simulink model "basic_control_structure_kalman"  (Simulink 6.2)
settings: Solver=ode45  StartTime=0.0  StopTime=6174  RelTol=1e-3
libraries: components_lib x12, simulink x5
settings Model: Creator=krage  LastModifiedBy=Martin  ExtModeAutoUpdateStatusClock=off
settings DebuggingCC: CheckSSInitialOutputMsg=off  SolverPrmCheckMsg=warning

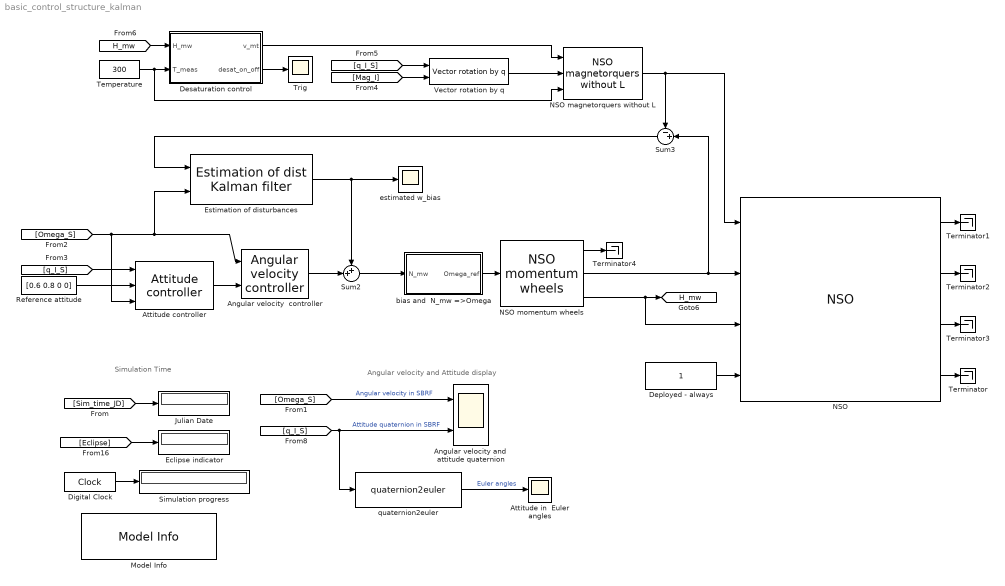
== system basic_control_structure_kalman ==
  note: Simulation Time
  note: Angular velocity and Attitude display
  Angular velocity  controller : components_lib/ACS/Controllers/Angular velocity  controller  ang_file_name='ang_robust_control.m'
  Angular velocity and  attitude quaternion : Scope  NumInputPorts=2
      settings: TimeRange=250  YMin=-0.05~0.1  YMax=0.05~0.9  SaveName=measurement
  Attitude controller : components_lib/ACS/Controllers/Attitude controller  att_file_name='attitude_control_lqr.m'
  Attitude in  Euler angles : Scope
      settings: YMin=-3.5  YMax=3.5
  Deployed - always : Constant
  Desaturation control : Subsystem  mask{h_bias=2.23*1e-3, desat_on=0.7*2.23e-3, desat_off=0.01*2.23e-3}
      mask prompts: h_bias "Angular momentum bias"; desat_on "Threshold desaturation on"; desat_off "Threshold desaturation off"
  Digital Clock : DigitalClock
  Eclipse indicator : Display
  Estimation of disturbances : components_lib/ACS/Controllers/Estimation of dist Kalman filter  ang_file_name='kalman_estimator.m'
  Julian Date : Display
  Model Info : simulink/Model-Wide Utilities/Model Info  InitialBlockCM=None  BlockCM=None  Frame=on  DisplayStringWithTags=|  HorizontalTextAlignment=Left  LeftAlignmentValue=0.02  SourceBlockDiagram=basic_control_structure_kalman  TagMaxNumber=20
      | Usefull Julian dates:
      | sun to eclipse : 2452315.560376
      | 32 sec. before : 2452315.56
      | eclipse to sun : 2452315.513363
  NSO : components_lib/NSO  Tag=AAUSAT-II Model  Description=AAUSAT-II Model  r_com_s=[0.05 0.05 0.15]  sat_temp_start=0  r_com_s_deployed=[0.05 0.05 0.125]  mass_sc=3  Dim=[0.1 0.1 0.3]  inertia_c=[25 25 5]/1e3  inertia_d=[42.3 42.3 28.4]/1e3  init_jd=2452315.56  q_s_c=[0 0 0 1]  q_init_s_i=[0.6 0.8 0 0]  w_init_s=[0.0021 -0.0021 0.0021]*0  Cd=2  rho=9.25e-13  enable_sensor_emulation=off  alb_emu_enabled=off  enable_dist=on
  NSO magnetorquers without L : components_lib/Actuator Emulation/NSO magnetorquers without L
  NSO momentum wheels : components_lib/Actuator Emulation/NSO momentum wheels  w_mw_i=[1078.6 1078.6 1078.6] *0.5
  Reference attitude : Constant  Value=[0.6 0.8 0 0]
  Simulation progress : Display
  Sum2 : Sum  Inputs=++|
  Sum3 : Sum  Orientation=left  Inputs=-+|
  Temperature : Constant  Value=300
  Terminator{,1..4} (5 alike) : Terminator
  Trig : Scope
      settings: YMin=0.95  YMax=1.05  SaveName=ScopeData2
  Vector rotation by q : components_lib/Math utilities/Quaternion operations/Vector rotation by q
  bias and  N_mw =>Omega : Subsystem
  estimated w_bias : Scope
      settings: TimeRange=6174  YMin=-5e-08  YMax=6e-08  SaveName=omega_est
  quaternion2euler : components_lib/Math utilities/Quaternion operations/quaternion2euler
  tag scope: H_mw=global
  wires:
  [Omega_S] -> Angular velocity and  attitude quaternion/1  "Angular velocity in SBRF"
  [q_I_S] -> quaternion2euler/1, Angular velocity and  attitude quaternion/2  "Attitude quaternion in SBRF"
  quaternion2euler/1 -> Attitude in  Euler angles/1  "Euler angles"
  [Sim_time_JD] -> Julian Date/1
  [Eclipse] -> Eclipse indicator/1
  Digital Clock/1 -> Simulation progress/1
  Deployed - always/1 -> NSO/4
  Angular velocity  controller/1 -> Sum2/2
  [Omega_S] -> Estimation of disturbances/2, Angular velocity  controller/1, Attitude controller/3
  Reference attitude/1 -> Attitude controller/2
  [q_I_S] -> Attitude controller/1
  NSO/1 -> Terminator1/1
  NSO/2 -> Terminator2/1
  NSO/3 -> Terminator3/1
  NSO/4 -> Terminator/1
  Estimation of disturbances/1 -> estimated w_bias/1, Sum2/1
  Attitude controller/1 -> Angular velocity  controller/2
  Temperature/1 -> NSO magnetorquers without L/3, Desaturation control/2(T_meas)
  bias and  N_mw =>Omega/1(Omega_ref) -> NSO momentum wheels/1
  Sum2/1 -> bias and  N_mw =>Omega/1(N_mw)
  [Mag_I] -> Vector rotation by q/2
  [q_I_S] -> Vector rotation by q/1
  Vector rotation by q/1 -> NSO magnetorquers without L/2
  Desaturation control/1(v_mt) -> NSO magnetorquers without L/1
  [H_mw] -> Desaturation control/1(H_mw)
  Desaturation control/2(desat_on_off) -> Trig/1
  NSO momentum wheels/3 -> [H_mw], NSO/3
  NSO momentum wheels/2 -> NSO/2, Sum3/2
  NSO momentum wheels/1 -> Terminator4/1
  NSO magnetorquers without L/1 -> Sum3/1, NSO/1
  Sum3/1 -> Estimation of disturbances/1

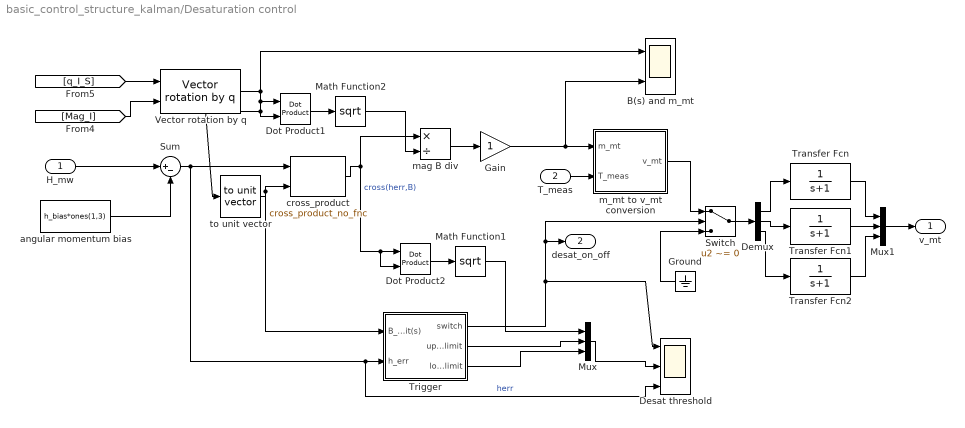
== system basic_control_structure_kalman/Desaturation control ==
  H_mw : Inport  Port=1  LatchInput=off
  T_meas : Inport  Port=2  LatchInput=off
  B(s) and m_mt : Scope  NumInputPorts=2
      settings: YMin=-2e-005~-1  YMax=2e-005~11  SaveName=ScopeData6
  Demux : Demux  Outputs=3
  Desat threshold : Scope  NumInputPorts=3
      settings: YMin=0~0~-0.0025  YMax=1~0.004~0.0025  SaveName=desat_info
  Dot Product1 : simulink/Math Operations/Dot Product  InputSameDT=on  OutDataType=sfix(16)  OutScaling=2^-10  DoSatur=off
  Dot Product2 : simulink/Math Operations/Dot Product  InputSameDT=on  OutDataType=sfix(16)  OutScaling=2^-10  DoSatur=off
  Gain : Gain
  Ground : Ground  Orientation=left
  Math Function1 : Math  Operator=sqrt  SaturateOnIntegerOverflow=on
  Math Function2 : Math  Operator=sqrt  SaturateOnIntegerOverflow=on
  Mux : Mux  Inputs=3
  Mux1 : Mux  Inputs=3
  Sum : Sum  Inputs=|+-
  Switch : Switch  Criteria=u2 ~= 0  Threshold=0.5
  Transfer Fcn : TransferFcn  Denominator=[1 1]
  Transfer Fcn1 : TransferFcn  Denominator=[1 1]
  Transfer Fcn2 : TransferFcn  Denominator=[1 1]
  Trigger : Subsystem
  Vector rotation by q : components_lib/Math utilities/Quaternion operations/Vector rotation by q
  angular momentum bias : Constant  Value=h_bias*ones(1,3)
  cross_product : components_lib/Math utilities/Vector operations/cross_product_no_fnc
  m_mt to v_mt conversion : Subsystem  mask{n_mt=[435 435 865], A_mt=[0.21*0.07 0.21*0.07 0.07*0.07], L_mt=[26.956e-3 26.956e-3 59.256e-3], v_max_mt=5}
      mask prompts: n_mt "Coil winding number [n_x n_y n_z]"; A_mt "Coil area [A_mt_x A_mt_y A_mt_z]"; L_mt "Coil inductance [L_mt_x L_mt_y L_mt_z]"; v_max_mt "Maximum voltage"
  mag B div : Product  Inputs=*/  OutScaling=2^-10
  to unit vector : components_lib/Math utilities/Vector operations/to unit vector
  v_mt : Outport
  desat_on_off : Outport  Port=2
  wires:
  H_mw/1 -> Sum/1
  angular momentum bias/1 -> Sum/2
  [Mag_I] -> Vector rotation by q/2
  [q_I_S] -> Vector rotation by q/1
  Sum/1 -> cross_product/1, Trigger/2(h_err), Desat threshold/3  "herr"
  Vector rotation by q/1 -> Dot Product1/1, Dot Product1/2, to unit vector/1, B(s) and m_mt/1
  cross_product/1 -> mag B div/1, Dot Product2/1, Dot Product2/2  "cross(herr,B)"
  Ground/1 -> Switch/3
  T_meas/1 -> m_mt to v_mt conversion/2(T_meas)
  mag B div/1 -> Gain/1
  m_mt to v_mt conversion/1(v_mt) -> Switch/1
  Dot Product1/1 -> Math Function2/1
  Math Function2/1 -> mag B div/2
  Gain/1 -> m_mt to v_mt conversion/1(m_mt), B(s) and m_mt/2
  to unit vector/1 -> cross_product/2, Trigger/1(B_unit(s))
  Switch/1 -> Demux/1
  Demux/1 -> Transfer Fcn/1
  Demux/2 -> Transfer Fcn1/1
  Demux/3 -> Transfer Fcn2/1
  Transfer Fcn/1 -> Mux1/1
  Transfer Fcn1/1 -> Mux1/2
  Transfer Fcn2/1 -> Mux1/3
  Mux1/1 -> v_mt/1
  Mux/1 -> Desat threshold/2
  Trigger/1(switch) -> Desat threshold/1, desat_on_off/1, Switch/2
  Trigger/2(upper limit) -> Mux/2
  Dot Product2/1 -> Math Function1/1
  Math Function1/1 -> Mux/1
  Trigger/3(lower limit) -> Mux/3

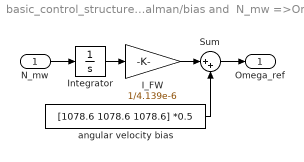
== system basic_control_structure_kalman/bias and  N_mw =>Omega ==
  N_mw : Inport  Port=1  LatchInput=off
  I_FW : Gain  Gain=1/4.139e-6
  Integrator : Integrator  InitialCondition=[2.23 2.23 2.23]*1e-3
  Sum : Sum  Inputs=|++
  angular velocity bias : Constant  Value=[1078.6 1078.6 1078.6] *0.5
  Omega_ref : Outport
  wires:
  I_FW/1 -> Sum/1
  angular velocity bias/1 -> Sum/2
  Integrator/1 -> I_FW/1
  N_mw/1 -> Integrator/1
  Sum/1 -> Omega_ref/1

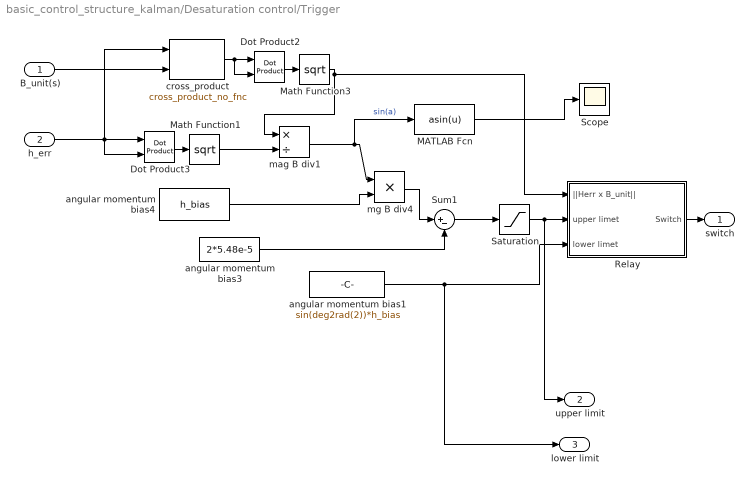
== system basic_control_structure_kalman/Desaturation control/Trigger ==
  B_unit(s) : Inport  Port=1  PortDimensions=3  LatchInput=off
  h_err : Inport  Port=2  LatchInput=off
  Dot Product2 : simulink/Math Operations/Dot Product  InputSameDT=on  OutDataType=sfix(16)  OutScaling=2^-10  DoSatur=off
  Dot Product3 : simulink/Math Operations/Dot Product  InputSameDT=on  OutDataType=sfix(16)  OutScaling=2^-10  DoSatur=off
  MATLAB Fcn : MATLABFcn  MATLABFcn=asin(u)
  Math Function1 : Math  Operator=sqrt  SaturateOnIntegerOverflow=on
  Math Function3 : Math  Operator=sqrt  SaturateOnIntegerOverflow=on
  Relay : Subsystem
  Saturation : Saturate  UpperLimit=inf  LowerLimit=2*sin(deg2rad(2))*h_bias
  Scope : Scope
      settings: YMin=0.5  YMax=1.6  SaveName=ScopeData4
  Sum1 : Sum  Inputs=|+-
  angular momentum bias1 : Constant  Value=sin(deg2rad(2))*h_bias
  angular momentum bias3 : Constant  Value=2*5.48e-5
  angular momentum bias4 : Constant  Value=h_bias
  cross_product : components_lib/Math utilities/Vector operations/cross_product_no_fnc
  mag B div1 : Product  Inputs=*/  OutScaling=2^-10
  mg B div4 : Product  OutScaling=2^-10
  switch : Outport
  upper limit : Outport  Port=2
  lower limit : Outport  Port=3
  wires:
  angular momentum bias3/1 -> Sum1/2
  Relay/1(Switch) -> switch/1
  angular momentum bias4/1 -> mg B div4/2
  mg B div4/1 -> Sum1/1
  Dot Product2/1 -> Math Function3/1
  Dot Product3/1 -> Math Function1/1
  Math Function1/1 -> mag B div1/2
  Sum1/1 -> Saturation/1
  mag B div1/1 -> mg B div4/1, MATLAB Fcn/1  "sin(a)"
  h_err/1 -> Dot Product3/1, Dot Product3/2, cross_product/1
  B_unit(s)/1 -> cross_product/2
  cross_product/1 -> Dot Product2/1, Dot Product2/2
  Math Function3/1 -> mag B div1/1, Relay/1(||Herr x B_unit||)
  angular momentum bias1/1 -> Relay/3(lower limet), lower limit/1
  MATLAB Fcn/1 -> Scope/1
  Saturation/1 -> Relay/2(upper limet), upper limit/1

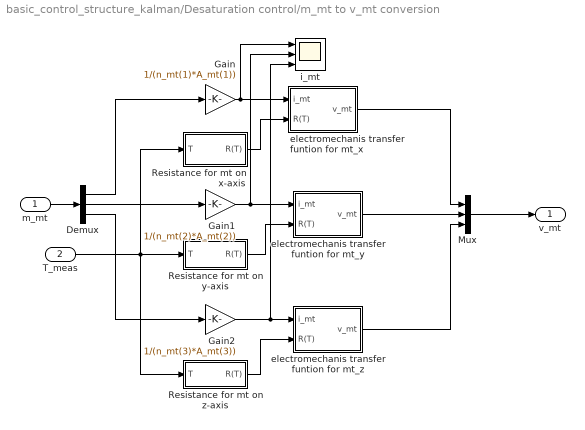
== system basic_control_structure_kalman/Desaturation control/m_mt to v_mt conversion ==
  m_mt : Inport  Port=1  LatchInput=off
  T_meas : Inport  Port=2  LatchInput=off
  Demux : Demux  Outputs=3
  Gain : Gain  Gain=1/(n_mt(1)*A_mt(1))
  Gain1 : Gain  Gain=1/(n_mt(2)*A_mt(2))
  Gain2 : Gain  Gain=1/(n_mt(3)*A_mt(3))
  Mux : Mux  Inputs=3
  Resistance for mt on x-axis : Subsystem  mask{A_wire_mt=(pi/4)*0.0002^2, sigma_0_mt=1.7e-8, alpha_0_mt=3.9e-3, T_0_mt=293}
      mask prompts: A_wire_mt "Wire cross sectional area"; sigma_0_mt "Wire resistivity"; alpha_0_mt "Wire resistivity temp. coef."; T_0_mt "Wire resistivity base temp."
  Resistance for mt on y-axis : Subsystem  mask{A_wire_mt=(pi/4)*0.0002^2, sigma_0_mt=1.7e-8, alpha_0_mt=3.9e-3, T_0_mt=293}
      mask prompts: A_wire_mt "Wire cross sectional area"; sigma_0_mt "Wire resistivity"; alpha_0_mt "Wire resistivity temp. coef."; T_0_mt "Wire resistivity base temp."
  Resistance for mt on z-axis : Subsystem  mask{A_wire_mt=(pi/4)*0.0002^2, sigma_0_mt=1.7e-8, alpha_0_mt=3.9e-3, T_0_mt=293}
      mask prompts: A_wire_mt "Wire cross sectional area"; sigma_0_mt "Wire resistivity"; alpha_0_mt "Wire resistivity temp. coef."; T_0_mt "Wire resistivity base temp."
  electromechanis transfer funtion for mt_x : Subsystem
  "electromechanis transfer funtion for mt_y " : Subsystem
  "electromechanis transfer funtion for mt_z " : Subsystem
  i_mt : Scope  NumInputPorts=3
      settings: YMin=-5~-5~-5  YMax=5~5~5  SaveName=ScopeData8
  v_mt : Outport
  wires:
  Demux/3 -> Gain2/1
  Demux/2 -> Gain1/1
  Demux/1 -> Gain/1
  Gain/1 -> electromechanis transfer funtion for mt_x/1(i_mt), i_mt/1
  Gain1/1 -> "electromechanis transfer funtion for mt_y "/1(i_mt), i_mt/2
  Gain2/1 -> "electromechanis transfer funtion for mt_z "/1(i_mt), i_mt/3
  m_mt/1 -> Demux/1
  "electromechanis transfer funtion for mt_y "/1(v_mt) -> Mux/2
  "electromechanis transfer funtion for mt_z "/1(v_mt) -> Mux/3
  Resistance for mt on x-axis/1(R(T)) -> electromechanis transfer funtion for mt_x/2(R(T))
  Resistance for mt on y-axis/1(R(T)) -> "electromechanis transfer funtion for mt_y "/2(R(T))
  Resistance for mt on z-axis/1(R(T)) -> "electromechanis transfer funtion for mt_z "/2(R(T))
  T_meas/1 -> Resistance for mt on y-axis/1(T), Resistance for mt on x-axis/1(T), Resistance for mt on z-axis/1(T)
  electromechanis transfer funtion for mt_x/1(v_mt) -> Mux/1
  Mux/1 -> v_mt/1

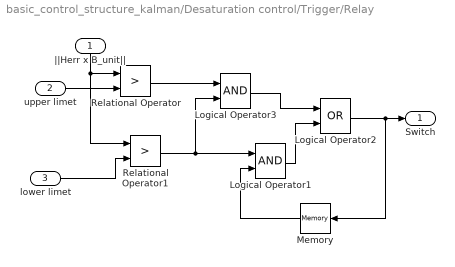
== system basic_control_structure_kalman/Desaturation control/Trigger/Relay ==
  ||Herr x B_unit|| : Inport  Orientation=down  Port=1  LatchInput=off
  upper limet : Inport  Port=2  LatchInput=off
  lower limet : Inport  Port=3  LatchInput=off
  Logical Operator1 : Logic  AllPortsSameDT=off  OutDataTypeMode=Boolean
  Logical Operator2 : Logic  Operator=OR  AllPortsSameDT=off  OutDataTypeMode=Boolean
  Logical Operator3 : Logic  AllPortsSameDT=off  OutDataTypeMode=Boolean
  Memory : Memory  Orientation=left
  Relational Operator : RelationalOperator  Operator=>  LogicOutDataTypeMode=Boolean  LogicDataType=1
  Relational Operator1 : RelationalOperator  Operator=>  LogicOutDataTypeMode=Boolean  LogicDataType=1
  Switch : Outport
  wires:
  ||Herr x B_unit||/1 -> Relational Operator/1, Relational Operator1/1
  Relational Operator1/1 -> Logical Operator1/1, Logical Operator3/2
  Logical Operator1/1 -> Logical Operator2/2
  Logical Operator2/1 -> Memory/1, Switch/1
  Memory/1 -> Logical Operator1/2
  upper limet/1 -> Relational Operator/2
  lower limet/1 -> Relational Operator1/2
  Relational Operator/1 -> Logical Operator3/1
  Logical Operator3/1 -> Logical Operator2/1

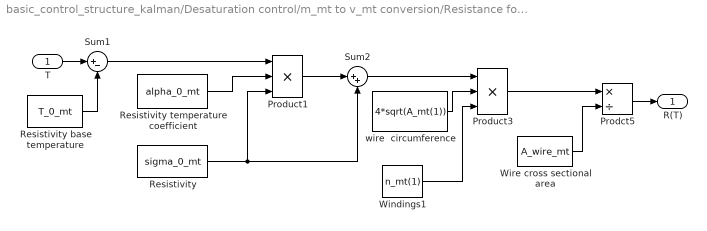
== system basic_control_structure_kalman/Desaturation control/m_mt to v_mt conversion/Resistance for mt on x-axis ==
  T : Inport  Port=1  LatchInput=off
  Prodct5 : Product  Inputs=*/  RndMeth=Zero
  Product1 : Product  Inputs=3  RndMeth=Zero
  Product3 : Product  Inputs=3  RndMeth=Zero
  Resistivity : Constant  Value=sigma_0_mt
  Resistivity base temperature : Constant  Value=T_0_mt
  Resistivity temperature coefficient : Constant  Value=alpha_0_mt
  Sum1 : Sum  Inputs=|+-
  Sum2 : Sum  Inputs=|++
  Windings1 : Constant  Value=n_mt(1)
  Wire cross sectional area : Constant  Value=A_wire_mt
  wire  circumference : Constant  Value=4*sqrt(A_mt(1))
  R(T) : Outport
  wires:
  Resistivity base temperature/1 -> Sum1/2
  Resistivity temperature coefficient/1 -> Product1/2
  Sum1/1 -> Product1/1
  Resistivity/1 -> Product1/3, Sum2/2
  Product1/1 -> Sum2/1
  Sum2/1 -> Product3/1
  wire  circumference/1 -> Product3/2
  Windings1/1 -> Product3/3
  Product3/1 -> Prodct5/1
  Wire cross sectional area/1 -> Prodct5/2
  T/1 -> Sum1/1
  Prodct5/1 -> R(T)/1

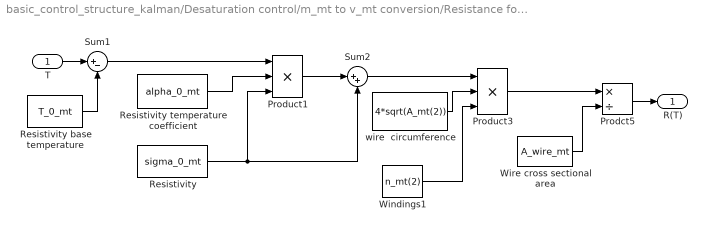
== system basic_control_structure_kalman/Desaturation control/m_mt to v_mt conversion/Resistance for mt on y-axis ==
  T : Inport  Port=1  LatchInput=off
  Prodct5 : Product  Inputs=*/  RndMeth=Zero
  Product1 : Product  Inputs=3  RndMeth=Zero
  Product3 : Product  Inputs=3  RndMeth=Zero
  Resistivity : Constant  Value=sigma_0_mt
  Resistivity base temperature : Constant  Value=T_0_mt
  Resistivity temperature coefficient : Constant  Value=alpha_0_mt
  Sum1 : Sum  Inputs=|+-
  Sum2 : Sum  Inputs=|++
  Windings1 : Constant  Value=n_mt(2)
  Wire cross sectional area : Constant  Value=A_wire_mt
  wire  circumference : Constant  Value=4*sqrt(A_mt(2))
  R(T) : Outport
  wires:
  Prodct5/1 -> R(T)/1
  T/1 -> Sum1/1
  Wire cross sectional area/1 -> Prodct5/2
  Product3/1 -> Prodct5/1
  Windings1/1 -> Product3/3
  wire  circumference/1 -> Product3/2
  Sum2/1 -> Product3/1
  Product1/1 -> Sum2/1
  Resistivity/1 -> Sum2/2, Product1/3
  Sum1/1 -> Product1/1
  Resistivity temperature coefficient/1 -> Product1/2
  Resistivity base temperature/1 -> Sum1/2

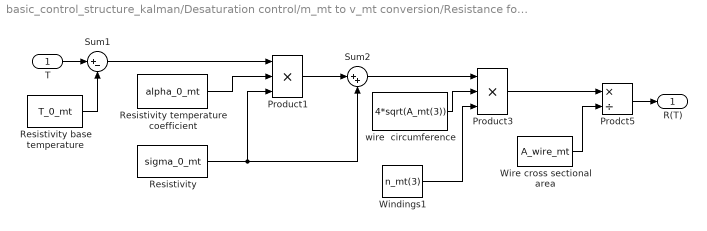
== system basic_control_structure_kalman/Desaturation control/m_mt to v_mt conversion/Resistance for mt on z-axis ==
  T : Inport  Port=1  LatchInput=off
  Prodct5 : Product  Inputs=*/  RndMeth=Zero
  Product1 : Product  Inputs=3  RndMeth=Zero
  Product3 : Product  Inputs=3  RndMeth=Zero
  Resistivity : Constant  Value=sigma_0_mt
  Resistivity base temperature : Constant  Value=T_0_mt
  Resistivity temperature coefficient : Constant  Value=alpha_0_mt
  Sum1 : Sum  Inputs=|+-
  Sum2 : Sum  Inputs=|++
  Windings1 : Constant  Value=n_mt(3)
  Wire cross sectional area : Constant  Value=A_wire_mt
  wire  circumference : Constant  Value=4*sqrt(A_mt(3))
  R(T) : Outport
  wires:
  Resistivity base temperature/1 -> Sum1/2
  Resistivity temperature coefficient/1 -> Product1/2
  Sum1/1 -> Product1/1
  Resistivity/1 -> Product1/3, Sum2/2
  Product1/1 -> Sum2/1
  Sum2/1 -> Product3/1
  wire  circumference/1 -> Product3/2
  Windings1/1 -> Product3/3
  Product3/1 -> Prodct5/1
  Wire cross sectional area/1 -> Prodct5/2
  T/1 -> Sum1/1
  Prodct5/1 -> R(T)/1

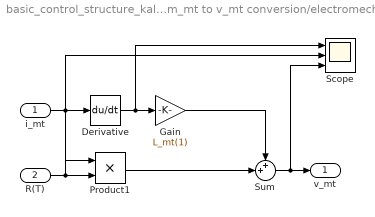
== system basic_control_structure_kalman/Desaturation control/m_mt to v_mt conversion/electromechanis transfer funtion for mt_x ==
  i_mt : Inport  Port=1  LatchInput=off
  R(T) : Inport  Port=2  LatchInput=off
  Derivative : Derivative
  Gain : Gain  Gain=L_mt(1)
  Product1 : Product  RndMeth=Zero
  Scope : Scope  NumInputPorts=3
      settings: YMin=-5~-5~-5  YMax=5~5~5  SaveName=ScopeData9
  Sum : Sum  Inputs=++|
  v_mt : Outport
  wires:
  Derivative/1 -> Gain/1, Scope/1
  Sum/1 -> v_mt/1, Scope/3
  i_mt/1 -> Derivative/1, Product1/1
  R(T)/1 -> Product1/2, Scope/2
  Product1/1 -> Sum/2
  Gain/1 -> Sum/1

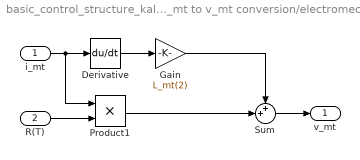
== system basic_control_structure_kalman/Desaturation control/m_mt to v_mt conversion/electromechanis transfer funtion for mt_y  ==
  i_mt : Inport  Port=1  LatchInput=off
  R(T) : Inport  Port=2  LatchInput=off
  Derivative : Derivative
  Gain : Gain  Gain=L_mt(2)
  Product1 : Product  RndMeth=Zero
  Sum : Sum  Inputs=++|
  v_mt : Outport
  wires:
  Gain/1 -> Sum/1
  Product1/1 -> Sum/2
  R(T)/1 -> Product1/2
  i_mt/1 -> Product1/1, Derivative/1
  Sum/1 -> v_mt/1
  Derivative/1 -> Gain/1

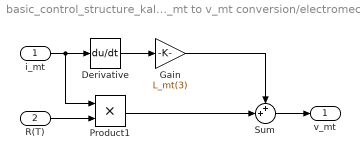
== system basic_control_structure_kalman/Desaturation control/m_mt to v_mt conversion/electromechanis transfer funtion for mt_z  ==
  i_mt : Inport  Port=1  LatchInput=off
  R(T) : Inport  Port=2  LatchInput=off
  Derivative : Derivative
  Gain : Gain  Gain=L_mt(3)
  Product1 : Product  RndMeth=Zero
  Sum : Sum  Inputs=++|
  v_mt : Outport
  wires:
  Derivative/1 -> Gain/1
  Sum/1 -> v_mt/1
  i_mt/1 -> Derivative/1, Product1/1
  R(T)/1 -> Product1/2
  Product1/1 -> Sum/2
  Gain/1 -> Sum/1
